simulink model "Fcn"  (R2015a)
settings: Solver=ode3  StartTime=0.0  StopTime=10.0  RelTol=1e-3
settings Model: Creator=hamza  LastModifiedBy=Teme
settings DataIOCC: LimitDataPoints=off  SaveFormat=Dataset
settings HardwareCC: ProdBitPerInt=16  ProdBitPerPointer=16  ProdIntDivRoundTo=Zero  ProdEndianess=LittleEndian  ProdWordSize=8  ProdShiftRightIntArith=off  ProdHWDeviceType=Intel->8051 Compatible  TargetBitPerInt=16  TargetBitPerPointer=16  TargetShiftRightIntArith=off  TargetIntDivRoundTo=Zero  TargetEndianess=LittleEndian  TargetWordSize=8  TargetHWDeviceType=Intel->8051 Compatible  ProdEqTarget=off
settings ModelReferenceCC: PropagateSignalLabelsOutOfModel=on
settings ConfigComp: CovMetricSettings=dw  CovHtmlReporting=on  CovSaveCumulativeToWorkspaceVar=on  CovSaveSingleToWorkspaceVar=on  CovExternalEMLEnable=off

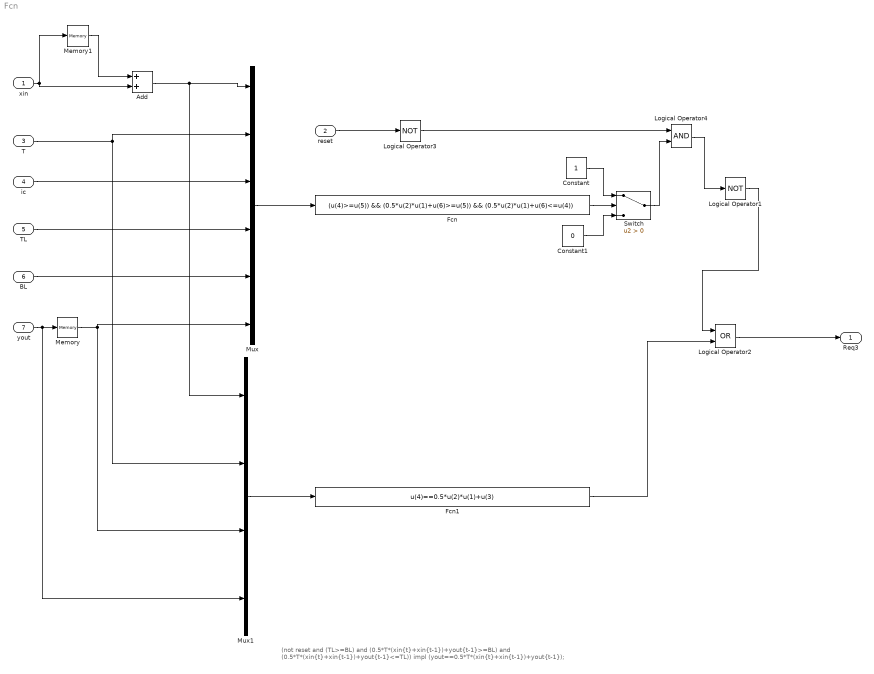
== system Fcn ==
  note: (not reset and (TL>=BL) and (0.5*T*(xin{t}+xin{t-1})+yout{t-1}>=BL) and (0.5*T*(xin{t}+xin{t-1})+yout{t-1}<=TL))
      | impl (yout==0.5*T*(xin{t}+xin{t-1})+yout{t-1});
  xin : Inport
  reset : Inport  Port=2
  T : Inport  Port=3
  ic : Inport  Port=4
  TL : Inport  Port=5
  BL : Inport  Port=6
  yout : Inport  Port=7
  Add : Sum
  Constant : Constant  OutDataTypeStr=boolean
  Constant1 : Constant  Value=0  OutDataTypeStr=boolean
  Fcn : Fcn  Expr=(u(4)>=u(5)) && (0.5*u(2)*u(1)+u(6)>=u(5)) && (0.5*u(2)*u(1)+u(6)<=u(4))
  Fcn1 : Fcn  Expr=u(4)==0.5*u(2)*u(1)+u(3)
  Logical Operator1 : Logic  Operator=NOT  AllPortsSameDT=off  OutDataTypeStr=boolean
  Logical Operator2 : Logic  Operator=OR  AllPortsSameDT=off  OutDataTypeStr=boolean
  Logical Operator3 : Logic  Operator=NOT  AllPortsSameDT=off  OutDataTypeStr=boolean
  Logical Operator4 : Logic  AllPortsSameDT=off  OutDataTypeStr=boolean
  Memory : Memory
  Memory1 : Memory
  Mux : Mux  Inputs=6
  Mux1 : Mux
  Switch : Switch  Criteria=u2 > Threshold
  Req3 : Outport
  wires:
  xin/1 -> Add/2, Memory1/1
  reset/1 -> Logical Operator3/1
  T/1 -> Mux/2, Mux1/2
  ic/1 -> Mux/3
  TL/1 -> Mux/4
  BL/1 -> Mux/5
  Mux/1 -> Fcn/1
  Fcn/1 -> Switch/2
  Memory1/1 -> Add/1
  Add/1 -> Mux1/1, Mux/1
  Logical Operator1/1 -> Logical Operator2/1
  Logical Operator2/1 -> Req3/1
  Fcn1/1 -> Logical Operator2/2
  yout/1 -> Mux1/4, Memory/1
  Mux1/1 -> Fcn1/1
  Memory/1 -> Mux1/3, Mux/6
  Logical Operator3/1 -> Logical Operator4/1
  Logical Operator4/1 -> Logical Operator1/1
  Switch/1 -> Logical Operator4/2
  Constant/1 -> Switch/1
  Constant1/1 -> Switch/3
